simulink model "Sim_Integrada"  (R2018a)
settings: Solver=ode15s  StartTime=0.0  StopTime=2  FixedStep=1e-3  MaxStep=0.1  RelTol=1e-4  AbsTol=1e-5  EnableMultiTasking=on
StartFcn:
  | tic;
StopFcn:
  | Elapsed_Sim_Time = toc;
  | disp(['Elapsed Sim Time = ' num2str(Elapsed_Sim_Time)]);
model workspace (MATLAB code in the model file):
  | whl.rad = 0.025;
  | whl.thickness = 0.005;
  | 
  | axle.length = 0.2;
  | axle.radius = 0.005;
  | platform.radius = 0.15;
  | platform.thickness = 0.005;
  | platform.offset = -0.01;
  | 
  | bumper.rad = platform.offset+whl.rad;
  | 
  | 
  | 
  | table.length = 1;
  | table.thickness = 0.01;
  | tableWhl.contact.k = 1e3;
  | tableWhl.contact.b = 1e2;
  | 
  | steel.density = 8000; %kg/m^3
  | 
  | start_pos.x = -0.2;
  | start_pos.y = 0.2;
  | 
  | l_whl_trq = [0 0 0 0.5 0 0 0 -0.5 1.0 0 0 0 -1.0 0.5 0 0 0 -0.5 -1.5 0 0 0 1.5].'*0.0005;
  | r_whl_trq = [0 0 0 2.0 0 0 0 -2.0 1.0 0 0 0 -1.0 1.0 0 0 0 -1.0 -1.5 0 0 0 1.5].'*0.0005;
undefined symbols (not defined in the file): X, Y, Z
libraries: sm_lib x60, fl_lib x38, nesl_utility x15, elec_lib x11, simulink x4, Contact_Forces_Lib x4
(part 3 of 3)

== system Sim_Integrada/Estrutura/Suporte Frontal ==
  Rigid Transform : sm_lib/Frames and Transforms/Rigid Transform  TranslationMethod=Cartesian  TranslationStandardOffset=0  TranslationLengthUnit=mm  TranslationStandardAxis=+Z  TranslationCartesianOffset=[-58/2 17/2 -19.4]  TranslationROffset=0  TranslationROffsetUnits=m  TranslationZOffset=0  TranslationZOffsetUnits=m  TranslationThetaOffset=0  TranslationThetaOffsetUnits=deg  RotationMethod=RotationSequence  RotationAngleUnits=deg  RotationStandardAxis=+X  RotationAngle=90  RotationArbitraryAxis=[0 0 1]  FollAlignAxisA=+X  BaseAlignAxisA=+Y  FollAlignAxisB=+Y  BaseAlignAxisB=+Z  RotationSequenceAxes=BaseAxes  RotationSequence=XZX  RotationSequenceAngles=[90 90 0]  RotationSequenceAnglesUnits=deg  RotationMatrix=[1 0 0; 0 1 0; 0 0 1]
  Rigid Transform2 : sm_lib/Frames and Transforms/Rigid Transform  TranslationMethod=Cartesian  TranslationStandardOffset=0  TranslationLengthUnit=mm  TranslationStandardAxis=+Z  TranslationCartesianOffset="[ -17/2 7.2  58/2]"  TranslationROffset=0  TranslationROffsetUnits=m  TranslationZOffset=0  TranslationZOffsetUnits=m  TranslationThetaOffset=0  TranslationThetaOffsetUnits=deg  RotationMethod=RotationSequence  RotationAngleUnits=deg  RotationStandardAxis=+X  RotationAngle=-90  RotationArbitraryAxis=[0 0 1]  FollAlignAxisA=+X  BaseAlignAxisA=+Y  FollAlignAxisB=+Y  BaseAlignAxisB=+Z  RotationSequenceAxes=BaseAxes  RotationSequence=YZY  RotationSequenceAngles=[-90 -90 0]  RotationSequenceAnglesUnits=deg  RotationMatrix=[1 0 0; 0 1 0; 0 0 1]
  Solid1 : sm_lib/Body Elements/Solid  InertiaType=CalculateFromGeometry  Mass=Massa  MassUnits=g  CenterOfMass=[0 0 0]  CenterOfMassUnits=m  MomentsOfInertia=[1 1 1]  MomentsOfInertiaUnits=kg*m^2  ProductsOfInertia=[0 0 0]  ProductsOfInertiaUnits=kg*m^2  DensityBased=off  Density=1000  DensityUnits=kg/m^3  DoExposeReferenceFrame=on  SerializedFrames=<Frames/>  GraphicType=FromGeometry  MarkerShape=Sphere  MarkerSize=10  GraphicVisPropType=SimpleVisualProperties  GraphicDiffuseColor=Cor  GraphicSpecularColor=[0.5 0.5 0.5 1.0]  GraphicAmbientColor=[0.15 0.15 0.15 1.0]  GraphicEmissiveColor=[0.0 0.0 0.0 1.0]  GraphicShininess=75  GraphicOpacity=1.0  GeometryShape=FromFile  RectangleSize=[1 1]  RectangleSizeUnits=m  BrickDimensions=[1 1 1]  BrickDimensionUnits=m  CylinderRadius=1  CylinderRadiusUnits=m  CylinderLength=1  CylinderLengthUnits=m  SphereRadius=1  SphereRadiusUnits=m  EllipsoidRadii=[1 1 1]  EllipsoidRadiiUnits=m  ExtrusionCrossSection=[1 1; -1 1; -1 -1; 1 -1]  ExtrusionCrossSectionUnits=m  ExtrusionLength=1  ExtrusionLengthUnits=m  PolygonNumSides=3  PolygonOuterRadius=1  PolygonOuterRadiusUnits=m  ExtGeomFileType=STEP  ExtGeomFileName=D:\Trabalho\IC VSSS\Robô Red\Estrutura\STEP Simulink\Suporte lateral.stp  ExtGeomFileUnits=m  RevolutionCrossSection=[1 1; 1 -1; 2 -1; 2 1]  RevolutionCrossSectionUnits=m  RevolutionExtent=Full  RevolutionAngle=180  RevolutionAngleUnits=deg
  Conn1 : PMIOPort  Side=Left
  Conn3 : PMIOPort  Port=2  Side=Right
  connections:
  Solid1/RConn1 -- Rigid Transform2/LConn1 -- Rigid Transform/RConn1
  Rigid Transform/LConn1 -- Conn1/RConn1
  Rigid Transform2/RConn1 -- Conn3/RConn1

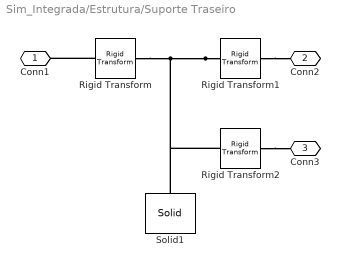
== system Sim_Integrada/Estrutura/Suporte Traseiro ==
  Rigid Transform : sm_lib/Frames and Transforms/Rigid Transform  TranslationMethod=Cartesian  TranslationStandardOffset=0  TranslationLengthUnit=mm  TranslationStandardAxis=+Z  TranslationCartesianOffset=[58/2 -17/2 -19.4]  TranslationROffset=0  TranslationROffsetUnits=m  TranslationZOffset=0  TranslationZOffsetUnits=m  TranslationThetaOffset=0  TranslationThetaOffsetUnits=deg  RotationMethod=RotationSequence  RotationAngleUnits=deg  RotationStandardAxis=+X  RotationAngle=90  RotationArbitraryAxis=[0 0 1]  FollAlignAxisA=+X  BaseAlignAxisA=+Y  FollAlignAxisB=+Y  BaseAlignAxisB=+Z  RotationSequenceAxes=BaseAxes  RotationSequence=XZX  RotationSequenceAngles=[90 -90 0]  RotationSequenceAnglesUnits=deg  RotationMatrix=[1 0 0; 0 1 0; 0 0 1]
  Rigid Transform1 : sm_lib/Frames and Transforms/Rigid Transform  TranslationMethod=Cartesian  TranslationStandardOffset=0  TranslationLengthUnit=mm  TranslationStandardAxis=+Z  TranslationCartesianOffset=[ -17/2 0 58/2]  TranslationROffset=0  TranslationROffsetUnits=m  TranslationZOffset=0  TranslationZOffsetUnits=m  TranslationThetaOffset=0  TranslationThetaOffsetUnits=deg  RotationMethod=RotationSequence  RotationAngleUnits=deg  RotationStandardAxis=+X  RotationAngle=-90  RotationArbitraryAxis=[0 0 1]  FollAlignAxisA=+X  BaseAlignAxisA=+Y  FollAlignAxisB=+Y  BaseAlignAxisB=+Z  RotationSequenceAxes=BaseAxes  RotationSequence=XYX  RotationSequenceAngles=[-90 90 0]  RotationSequenceAnglesUnits=deg  RotationMatrix=[1 0 0; 0 1 0; 0 0 1]
  Rigid Transform2 : sm_lib/Frames and Transforms/Rigid Transform  TranslationMethod=Cartesian  TranslationStandardOffset=0  TranslationLengthUnit=mm  TranslationStandardAxis=+Z  TranslationCartesianOffset="[ -17/2 7.2  58/2]"  TranslationROffset=0  TranslationROffsetUnits=m  TranslationZOffset=0  TranslationZOffsetUnits=m  TranslationThetaOffset=0  TranslationThetaOffsetUnits=deg  RotationMethod=RotationSequence  RotationAngleUnits=deg  RotationStandardAxis=+X  RotationAngle=-90  RotationArbitraryAxis=[0 0 1]  FollAlignAxisA=+X  BaseAlignAxisA=+Y  FollAlignAxisB=+Y  BaseAlignAxisB=+Z  RotationSequenceAxes=BaseAxes  RotationSequence=YZY  RotationSequenceAngles=[-90 -90 0]  RotationSequenceAnglesUnits=deg  RotationMatrix=[1 0 0; 0 1 0; 0 0 1]
  Solid1 : sm_lib/Body Elements/Solid  InertiaType=CalculateFromGeometry  Mass=Massa  MassUnits=g  CenterOfMass=[0 0 0]  CenterOfMassUnits=m  MomentsOfInertia=[1 1 1]  MomentsOfInertiaUnits=kg*m^2  ProductsOfInertia=[0 0 0]  ProductsOfInertiaUnits=kg*m^2  DensityBased=off  Density=1000  DensityUnits=kg/m^3  DoExposeReferenceFrame=on  SerializedFrames=<Frames/>  GraphicType=FromGeometry  MarkerShape=Sphere  MarkerSize=10  GraphicVisPropType=SimpleVisualProperties  GraphicDiffuseColor=Cor  GraphicSpecularColor=[0.5 0.5 0.5 1.0]  GraphicAmbientColor=[0.15 0.15 0.15 1.0]  GraphicEmissiveColor=[0.0 0.0 0.0 1.0]  GraphicShininess=75  GraphicOpacity=1.0  GeometryShape=FromFile  RectangleSize=[1 1]  RectangleSizeUnits=m  BrickDimensions=[1 1 1]  BrickDimensionUnits=m  CylinderRadius=1  CylinderRadiusUnits=m  CylinderLength=1  CylinderLengthUnits=m  SphereRadius=1  SphereRadiusUnits=m  EllipsoidRadii=[1 1 1]  EllipsoidRadiiUnits=m  ExtrusionCrossSection=[1 1; -1 1; -1 -1; 1 -1]  ExtrusionCrossSectionUnits=m  ExtrusionLength=1  ExtrusionLengthUnits=m  PolygonNumSides=3  PolygonOuterRadius=1  PolygonOuterRadiusUnits=m  ExtGeomFileType=STEP  ExtGeomFileName=D:\Trabalho\IC VSSS\Robô Red\Estrutura\STEP Simulink\Suporte lateral.stp  ExtGeomFileUnits=m  RevolutionCrossSection=[1 1; 1 -1; 2 -1; 2 1]  RevolutionCrossSectionUnits=m  RevolutionExtent=Full  RevolutionAngle=180  RevolutionAngleUnits=deg
  Conn1 : PMIOPort  Side=Left
  Conn2 : PMIOPort  Port=2  Side=Right
  Conn3 : PMIOPort  Port=3  Side=Right
  connections:
  Rigid Transform1/RConn1 -- Conn2/RConn1
  Rigid Transform1/LConn1 -- Rigid Transform2/LConn1 -- Solid1/RConn1 -- Rigid Transform/RConn1
  Rigid Transform/LConn1 -- Conn1/RConn1
  Rigid Transform2/RConn1 -- Conn3/RConn1

== matlab function Sim_Integrada/Dinâmica/MCU ==
  settings: updateMethod=DISCRETE  sampleTime=1e-4
  data: encAM1 input; encBM1 input; encAM2 input; encBM2 input; vtarget input; clock input; acaoM1 output; acaoM2 output; velM1 output; velM2 output
function [acaoM1, acaoM2,velM1,velM2] = fcn(encAM1,encBM1,encAM2,encBM2, vtarget,clock)
persistent t0
persistent encSM1_P
persistent encSM2_P
persistent periodo0
persistent erro1M1
persistent erro2M1
persistent erro1M2
persistent erro2M2
persistent acao1M1
persistent acao1M2
persistent clock_p
persistent velM1_p
persistent velM2_p
% ##############################################
%Inicialização das variáveis persistentes

if isempty(clock_p)
    clock_p = clock;
end
if isempty(t0)
    t0 = 0;
end
if isempty(encSM1_P)
    encSM1_P = 0.0;
end
if isempty(encSM2_P)
    encSM2_P = 0.0;
end
if isempty(periodo0)
    periodo0 = 0.0;
end   
if isempty(erro1M1)
    erro1M1 = vtarget;
end

if isempty(erro2M1)
    erro2M1 = vtarget;
end
if isempty(acao1M1)
    acao1M1 = 0;
end

if isempty(erro1M2)
    erro1M2 = vtarget;
end

if isempty(erro2M2)
    erro2M2 = vtarget;
end
if isempty(acao1M2)
    acao1M2 = 0;
end


if isempty(velM1_p)
    velM1_p = 0;
end
if isempty(velM2_p)
    velM2_p = 0;
end
% ##############################################

% Parametros de controle da velocidade
T = 1e-2; % Tempo de discretização de 10ms
npulsos = 12;

K1 = 100;
Td1 = 1e-3;
Ti1 = 5e1;

K2 = 100;
Td2 = 1e-3;
Ti2 = 5e1;


% ##############################################

% Fusão dos sinais dos dois canais
encSM1 = encAM1 + encBM1;
encSM2 = encAM2 + encBM2;
% pulseM1 = encSM1;
% pulseM2 = encSM2;
% ##############################################

% Calculo da velociadade

% Fórmula para tempo de 10ms e redução de 100:1
if clock > clock_p
    clock_p  = clock;
    
    VelM1 = (pi*(encSM1-encSM1_P))/(npulsos);
    VelM2 = (pi*(encSM2-encSM2_P))/(npulsos);
    encSM1_P = encSM1;
    encSM2_P = encSM2;

    velM1 = VelM1;
    velM2 = VelM2;
    velM1_p = velM1;
    velM2_p = velM2;
    % ##############################################

    % Calculo da ação de controle

    erroM1 = vtarget - VelM1;

    erroM2 = vtarget - VelM2;

    acaoM1 = acao1M1 + K1*((1 + T/Ti1 + Td1/T)*erroM1 - (1 - 2*Td1/T)*erro1M1 + Td1/T*erro2M1);
    acaoM2 = acao1M2 + K2*((1 + T/Ti2 + Td2/T)*erroM2 - (1 - 2*Td2/T)*erro1M2 + Td2/T*erro2M2);
%     acaoM1 = acao1M1 + K1*erroM1 - Td1*erro1M1 + Ti1*erro2M1;
%     acaoM2 = acao1M2 + K2*erroM2 - Td2*erro1M2 + Ti2*erro2M2;
%     acaoM1 = acao1M1 + K1*erroM1;
%     acaoM2 = acao1M2 + K2*erroM2;

    if acaoM1 < 0
        acaoM1 = 0;
    end
    if acaoM1 > 3200
        acaoM1 = 3200;
    end
    if acaoM2 < 0
        acaoM2 = 0;
    end
    if acaoM2 > 3200
        acaoM2 = 3200;
    end
    erro2M1 = erro1M1;
    erro1M1 = erroM1;

    erro2M2 = erro1M2;
    erro1M2 = erroM2;
    
    acao1M1 = acaoM1;
    acao1M2 = acaoM2;
else
    acaoM1 = acao1M1;
    acaoM2 = acao1M2;
    velM1 = velM1_p;
    velM2 = velM2_p;
end

% ##############################################
